simulink model "ex4_s"  (R2018b)
settings: Solver=VariableStepAuto  StartTime=0.0  StopTime=30.0  RelTol=1e-3
values from neighbouring files (symbols this model uses):
  A = [-11 -2.5 0;4 0 0;0 0.25 0]    [ex1.m]    (also in ex2.m; ex3.m = sys_s.a; ex4.m = sys_s.A; ex5.m = sys_c.A)
  B = [4 0 0]'    [ex1.m]    (also in ex2.m; ex3.m = sys_s.b; ex4.m = sys_s.B; ex5.m = sys_c.B)
  C = [0 0 5]    [ex1.m]    (also in ex2.m; ex3.m = sys_s.c; ex4.m = sys_s.C; ex5.m = sys_c.C)
  k_d = 2    [ex2.m]    (also in ex3.m; ex4.m; ex5.m; ex6.m)
  k_i = Kt(4)    [ex4.m]    (also in ex5.m = T*Kt(4); ex6.m = T*Kt(4); motore_posizione.m)
  k_x = Kt(1:3)    [ex4.m]    (also in ex5.m; ex6.m; motore_posizione.m)
settings Model: Creator=michelemaresca  LastModifiedBy=michelemaresca

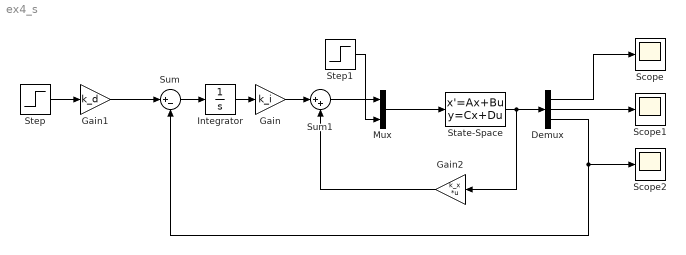
== system ex4_s ==
  Demux : Demux  Outputs=3
  Gain : Gain  Gain=k_i
  Gain1 : Gain  Gain=k_d
  Gain2 : Gain  Gain=k_x  Multiplication=Matrix(K*u)
  Integrator : Integrator
  Mux : Mux  Inputs=2
  Scope : Scope
  Scope1 : Scope
  Scope2 : Scope
  State-Space : StateSpace  A=A  B=[B,[0;0;1]]  C=[1 0 0;0 1 0;C]  D=zeros(3,2)  InitialCondition=0
  Step : Step  Time=0  SampleTime=0
  Step1 : Step  Time=10  After=40  SampleTime=0
  Sum : Sum  Inputs=|+-
  Sum1 : Sum  Inputs=|++
  wires:
  Integrator/1 -> Gain/1
  Sum/1 -> Integrator/1
  Step/1 -> Gain1/1
  Gain1/1 -> Sum/1
  Gain/1 -> Sum1/1
  Mux/1 -> State-Space/1
  Sum1/1 -> Mux/1
  Step1/1 -> Mux/2
  State-Space/1 -> Demux/1, Gain2/1
  Gain2/1 -> Sum1/2
  Demux/2 -> Scope1/1
  Demux/1 -> Scope/1
  Demux/3 -> Scope2/1, Sum/2
